simulink model "Backhoe_Arm_LS"  (R2013a)
settings: Solver=ode23t  StartTime=0.0  StopTime=30  MaxStep=0.01  RelTol=1e-3
PostLoadFcn:
  | warning off sm:compiler:state:UnsatisfiedDesiredTarget
  | warning off simscape:compiler:sli:init:SolverNotRecommended
  | warning off sm:sli:visualization:UnsupportedSimMode
  | warning off xPCTarget:sampleTime:sampleTimeInvariance
  | warning off sm:sli:setup:compile:LocalSolverNotSupported
model workspace (MAT data in the model file):
  cylinderGray = [0.6 0.6 0.6]
  darkOrange = [0.8 0.5 0]
  glassBlue = [0.2 0.2 1]
  gray = [0.3 0.3 0.3]
  orange = [0.8 0.65 0]
  pistonGray = [0.4 0.4 0.4]
  tireBlack = [0.1 0.1 0.1]
  wheelGray = [0.6 0.6 0.6]
  yellow = [0.8 0.8 0]
  rhoGlass = 2500
  rhoRubber = 1500
  rhoSteel = 7800
undefined symbols (not defined in the file or in its folder): BH_Param, sigbuilder_block, X, Y, Z
libraries: sm_lib x97, fl_lib x31, Backhoe_Lib x28, nesl_utility x21, sh_lib x9, xpclib x1
(part 1 of 4)
Description:
  | Copyright 2013 The MathWorks, Inc.
settings Model: ExtModeTrigDuration=3334  BufferReuse=off  Creator=smiller  LastModifiedBy=smiller
settings DataIOCC: LimitDataPoints=off
settings OptimizationCC: BlockReduction=off  OptimizeBlockIOStorage=off  BufferReuse=off  ExpressionFolding=off  ExpressionDepthLimit=2147483647  LocalBlockOutputs=off
settings DebuggingCC: SolverPrmCheckMsg=none
settings HardwareCC: ProdIntDivRoundTo=Zero  ProdEndianess=LittleEndian  ProdHWDeviceType=Generic->32-bit x86 compatible
settings RTWCC: SystemTargetFile=xpctarget.tlc  TemplateMakefile=xpc_default_tmf  Description=xPC Target  ProcessScript=xpctarget_make_rtw_hook  RTWCompilerOptimization=On
settings xpcTargetCC: TargetFcnLib=ansi_tfl_table_tmw.mat  CodeReplacementLibrary=XPC_BLAS  ParMdlRefBuildCompliant=on  ConcurrentExecutionCompliant=on  CombineSignalStateStructs=off  MATLABClassNameForMDSCustomization=xpcAperiodicCustomization  GRTInterface=on  GenerateAllocFcn=off  RL32LogBufSizeModifier=300000  xPCTaskExecutionProfile=off  xPCRL32EventNumber=5000  xPCLoadParamSetFile=off  xPCConcurrentTasks=off  xPCEnableSFAnimation=off
settings SimscapeCC: ExplicitSolverDiagnosticOptions=none
settings SimMechanicsCC: WarnOnRedundantConstraints=off
settings ExplorerConfigSet: InternalSimMechanicsExplorerSettings="<ExplorerConfiguration><canonicalview>default</canonicalview><TilePanel><TileInfo><Tiles Columns=\"1\" Count=\"1\" Rows=\"1\"><Column Left=\"2\" Weight=\"1\"/><Column Left=\"578\"/><Row Top=\"2\" Weight=\"1\"/><Row Top=\"405\"/><Tile Height=\"1\" Width=\"1\" X=\"0\" Y=\"0\"/></Tiles></TileInfo><SceneInfo><SceneViewer><BGColor><R>0.60000002384185791</R><G>0.60000002384185791</G><B>0.60000002384185791</B></BGColor><Camera><Position><X>19.674615884217218</X><Y>-11.790119899138375</Y><Z>8.3681328173355993</Z></Position><Center><X>1.1094029723013152</X><Y>-6.846774749183913</Y><Z>3.8240043455340573</Z></Center><Up><X>-0.20829119430312451</X><Y>0.11101192583651653</Y><Z>0.97174643333425503</Z></Up><Left>-4.3797052145004276</Left><Right>4.3797052145004276</Right><Bottom>-5.0912822484970093</Bottom><Top>5.0912822484970093</Top></Camera></SceneViewer></SceneInfo></TilePanel></ExplorerConfiguration>"

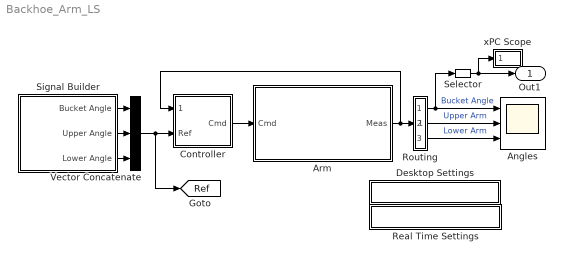
== system Backhoe_Arm_LS ==
  Angles : Scope  NumInputPorts=3
      settings: YMin=-120~-40~-70  YMax=20~60~-20
  Arm : Subsystem
      mask Display:
      | image(imread('Backhoe_Arm_IMAGE.JPG'));
      | port_label('input',1,'Cmd');
      | port_label('Output',1,'Meas');
  Controller : Subsystem
  Desktop Settings : Subsystem
      settings: OpenFcn=|
      | set_param(bdroot,'Solver','ODE23t','MaxStep','0.01','RelTol','1e-3','AbsTol','auto');
      | tvar_solverBlock = find_system(bdroot, 'SubClassName', 'solver');
      | 
      | for i=1:size(tvar_solverBlock,1)
      | 
      | set_param(char(tvar_solverBlock(i)), 'UseLocalSolver','off','DoFixedCost','off');
      | end
      | 
      | clear tvar_solverBlock
      mask Display: disp('Desktop Settings')
  Real Time Settings : Subsystem
      settings: OpenFcn=|
      | tvar_Nonlinear_Iterations = '2';
      | tvar_StepSize = '0.0004';                                                                                              %tvar_LocalSolver = 'NE_TRAPEZOIDAL_ADVANCER';
      | tvar_LocalSolver = 'NE_BACKWARD_EULER_ADVANCER';
      | set_param(bdroot,'Solver','ode1','FixedStep','auto');
      | tvar_solverBlock = find_system(bdroot, 'SubClassName', 'solver');
      | for i=1:size(tvar_solverBlock,1)
      | 
      | set_param(char(tvar_solverBlock(i)), 'UseLocalSolver','on','DoFixedCost','on','MaxNonlinIter',tvar_Nonlinear_Iterations,'LocalSolverChoice',tvar_LocalSolver,'LocalSolverSampleTime',tvar_StepSize);
      | end
      | clear tvar_Nonlinear_Iterations tvar_StepSize tvar_LocalSolver tvar_solverBlock
      mask Display: disp('Real Time Settings')
  Routing : Subsystem
  Selector : Selector  InputPortWidth=2  IndexOptions=Index vector (dialog)  Indices=[1]  OutputSizes=1
  Signal Builder : Subsystem  Tag=STV Subsys  LoadFcn=sigbuilder_block('load');  StartFcn=sigbuilder_block('start');  StopFcn=sigbuilder_block('stop');  ClipboardFcn=sigbuilder_block('clipboard');  mask(Sigbuilder block){}
      mask help: Simulink:masks:SigbuilderBlock_MD
      mask init:
      | if ~strcmp(get_param(bdroot(gcbh),'SimulationStatus'),'stopped') tuvar = sigbuilder_block('maskInit'); end
      settings: CopyFcn=sigbuilder_block('copy');  DeleteFcn=sigbuilder_block('delete');  ModelCloseFcn=sigbuilder_block('modelClose');  PreSaveFcn=sigbuilder_block('preSave');  PauseFcn=sigbuilder_block('pause');  ContinueFcn=sigbuilder_block('continue');  NameChangeFcn=sigbuilder_block('namechange');  OpenFcn=sigbuilder_block('open',[5.58621 7.44828 624.414 412.138 ]);  CloseFcn=sigbuilder_block('close');
      mask Display: plot(0, 0, 100, 100,[2, 2, 32, 32, 2], [68, 8, 8, 68, 68],[32, 2], [38, 38], [32, 19, 2],[53, 60, 44], [32, 17, 17, 2],[16, 16, 31, 31]);txt = getActiveGroup(gcbh);text(2, 100, txt,'verticalAlignment', 'top');
  Vector Concatenate : Concatenate  NumInputs=3
  xPC Scope : Subsystem
      mask Display: disp('xPC')
  Out1 : Outport
  tag scope: Ref=global
  wires:
  Signal Builder/2(Upper Angle) -> Vector Concatenate/2
  Signal Builder/1(Bucket Angle) -> Vector Concatenate/1
  Signal Builder/3(Lower Angle) -> Vector Concatenate/3
  Vector Concatenate/1 -> [Ref], Controller/2(Ref)
  Arm/1(Meas) -> Controller/1(Meas), Routing/1(Meas)
  Controller/1(Cmd) -> Arm/1(Cmd)
  Routing/2(UArm) -> Angles/2  "Upper Arm"
  Routing/3(LArm) -> Angles/3  "Lower Arm"
  Routing/1(Bucket) -> Angles/1, Selector/1  "Bucket Angle"
  Selector/1 -> xPC Scope/1(In1), Out1/1

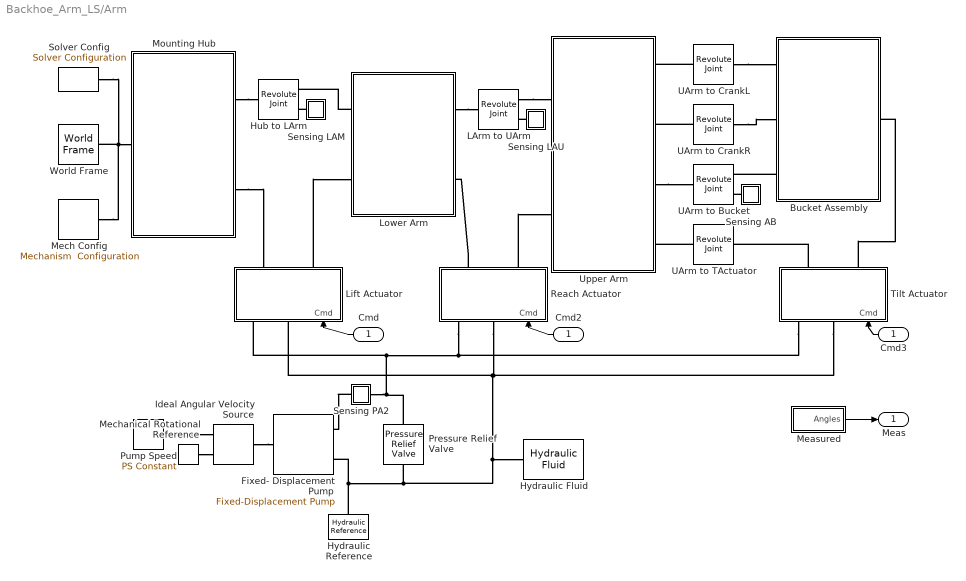
== system Backhoe_Arm_LS/Arm ==
  Cmd : Inport
  Bucket Assembly : Subsystem
      mask Display:
      | image(imread('Backhoe_Arm_Bucket_Asy_IMAGE.JPG'));
      | port_label('lconn',1,'UAL');
      | port_label('lconn',2,'UAR');
      | port_label('lconn',3,'UA');
      | port_label('rconn',1,'TAct');
  Cmd2 : InportShadow
  Cmd3 : InportShadow
  Fixed- Displacement Pump : sh_lib/Pumps and Motors/Fixed-Displacement Pump  D=BH_Param.Hydraulic.Pump.Displacement m^3/rad  efficiency_vol=BH_Param.Hydraulic.Pump.Vol_Eff  efficiency_tot=BH_Param.Hydraulic.Pump.Total_Eff  pr_nominal=BH_Param.Hydraulic.Pump.Nominal_Pressure Pa  w_nominal=BH_Param.Hydraulic.Pump.Nominal_Ang_Vel rad/s  visc_nominal=BH_Param.Hydraulic.Pump.Nominal_Kin_Visc cSt  pump_delivery_Log=off  leakage_flow_Log=off  torque_Log=off  power_hyd_Log=off  pressure_diff_Log=off  shaft_ang_vel_Log=off  LocalVarNames=|pump_delivery|leakage_flow|torque|power_hyd|pressure_diff|shaft_ang_vel  LocalVarDescs=|Pump delivery (m^3/s)|Leakage flow rate (m^3/s)|Driving shaft torque (N*m)|Output flow power (W)|Pressure differential (Pa)|Driving shaft angular velocity (rad/s)  LocalVarLogging=[0 0 0 0 0 0]
  Hub to LArm : sm_lib/Joints/Revolute Joint  SenseConstraintForceX=off  SenseConstraintForceY=off  SenseConstraintForceZ=off  SenseConstraintTorqueX=off  SenseConstraintTorqueY=off  SenseConstraintTorqueZ=off  ConstraintWrenchDir=FollowerOnBase  ConstraintWrenchFrame=BaseFrame  EquilibriumPosition=0  EquilibriumPositionUnits=deg  SpringStiffness=0  SpringStiffnessUnits=N*m/deg  DampingCoefficient=0  DampingCoefficientUnits=N*m/(deg/s)  ActuationMode=NoActuation  SensePosition=on  SenseVelocity=off  SenseAcceleration=off  SenseTorqueForce=off  PositionTargetValue=-60  PositionTargetValueUnits=deg  PositionTargetSpecify=on  PositionTargetPriority=High  VelocityTargetValue=0  VelocityTargetValueUnits=deg/s  VelocityTargetSpecify=off  VelocityTargetPriority=High  BlockFunction=simmechanics.library.joints.revolute_joint
  Hydraulic Reference : fl_lib/Hydraulic/Hydraulic Elements/Hydraulic Reference  q_Log=off  LocalVarNames=|q  LocalVarDescs=|q  LocalVarLogging=[]
  Hydraulic Fluid : sh_lib/Hydraulic Utilities/Hydraulic Fluid  Tag=Factory Generic  DataSource=1  SelFluid=9  SysTemp=50 c  TrapAir=0.004  ViscDerFactor=1  LocalVarLogging=[]
  Ideal Angular Velocity Source : fl_lib/Mechanical/Mechanical Sources/Ideal Angular Velocity Source  w_Log=off  t_Log=off  LocalVarNames=|torque|rel_velocity|power  LocalVarDescs=|Torque (N*m)|Relative velocity (rad/s)|Power generated by the sourcec(W)  LocalVarLogging=[0 0 0]
  LArm to UArm : sm_lib/Joints/Revolute Joint  SenseConstraintForceX=off  SenseConstraintForceY=off  SenseConstraintForceZ=off  SenseConstraintTorqueX=off  SenseConstraintTorqueY=off  SenseConstraintTorqueZ=off  ConstraintWrenchDir=FollowerOnBase  ConstraintWrenchFrame=BaseFrame  EquilibriumPosition=0  EquilibriumPositionUnits=deg  SpringStiffness=0  SpringStiffnessUnits=N*m/deg  DampingCoefficient=0  DampingCoefficientUnits=N*m/(deg/s)  ActuationMode=NoActuation  SensePosition=on  SenseVelocity=off  SenseAcceleration=off  SenseTorqueForce=off  PositionTargetValue=50  PositionTargetValueUnits=deg  PositionTargetSpecify=on  PositionTargetPriority=High  VelocityTargetValue=0  VelocityTargetValueUnits=deg/s  VelocityTargetSpecify=off  VelocityTargetPriority=High  BlockFunction=simmechanics.library.joints.revolute_joint
  Lift Actuator : Subsystem  mask(Hydraulic Actuator){Lcyl=BH_Param.Lift_Actuator.Cyl_Dims.Lcyl, Rcyl=BH_Param.Lift_Actuator.Cyl_Dims.Rcyl, Lbase=BH_Param.Lift_Actuator.Cyl_Dims.Lbase, Wbase=BH_Param.Lift_Actuator.Cyl_Dims.Wbase, Rbp=BH_Param.Lift_Actuator.Cyl_Dims.Rbp, Lbp=BH_Param.Lift_Actuator.Cyl_Dims.Lbp, Lpist=BH_Param.Lift_Actuator.Piston_Dims.Lpist, Rpist=BH_Param.Lift_Actuator.Piston_Dims.Rpist, Whead=BH_Param.Lift_Actuator.Piston_Dims.Whead, Lhead=BH_Param.Lift_Actuator.Piston_Dims.Lhead, Rhp=BH_Param.Lift_Actuator.Piston_Dims.Rhp, Lhp=BH_Param.Lift_Actuator.Piston_Dims.Lhp, hydr_area=BH_Param.Lift_Actuator.Cylinder.Area_A, hydr_stroke=BH_Param.Lift_Actuator.Cylinder.Stroke, hydr_deadvol=BH_Param.Lift_Actuator.Cylinder.DeadVol_A, hydr_x0=BH_Param.Lift_Actuator.Cylinder.x0, hydr_PA0=BH_Param.Lift_Actuator.Cylinder.PA0, hydr_PB0=BH_Param.Lift_Actuator.Cylinder.PB0, hydr_valve_max_area=BH_Param.Lift_Actuator.Valve.Max_Area, hydr_valve_max_opening=BH_Param.Lift_Actuator.Valve.Max_Opening, friction_breakaway=BH_Param.Lift_Actuator.Friction.Breakaway, friction_coulomb=BH_Param.Lift_Actuator.Friction.Coulomb, friction_viscous=BH_Param.Lift_Actuator.Friction.Viscous, circlePoints=25, cylColor=BH_Param.Colors.cylinderGray, rhoCyl=BH_Param.Densities.rhoSteel, pistColor=BH_Param.Colors.pistonGray, rhoPist=BH_Param.Densities.rhoSteel, connColor=BH_Param.Colors.gray, rhoConn=BH_Param.Densities.rhoSteel}
      mask prompts: Lcyl "Lcyl [m]"; Rcyl "Rcyl [m]"; Lbase "Lbase [m]"; Wbase "Wbase [m]"; Rbp "Rbp [m]"; Lbp "Lbp [m]"; Lpist "Lpist [m]"; Rpist "Rpist [m]"; Whead "Whead [m]"; Lhead "Lhead [m]"; Rhp "Rhp [m]"; Lhp "Lhp [m]"; hydr_area "Piston Area [m^3]"; hydr_stroke "Piston Stroke [m]"; hydr_deadvol "Dead Volume [m^3]"; hydr_x0 "Initial Position [m]"; hydr_PA0 "Initial Pressure, Chamber A [Pa]"; hydr_PB0 "Initial Pressure, Chamber B [Pa]"; hydr_valve_max_area "Valve Max Area [mm^2]"; hydr_valve_max_opening "Valve Max Opening [m]"; friction_breakaway "Breakaway Friction Force [N]"; friction_coulomb "Coulomb Friction Force [N]"; friction_viscous "Viscous Friction Coefficient [N/(m/2)]"; circlePoints "Circle Mesh Resolution"; cylColor "Cylinder Color"; rhoCyl "Cylinder Density [kg/m^3]"; pistColor "Piston Color"; rhoPist "Piston Density [kg/m^3]"; connColor "Connector Color"; rhoConn "Connector Density [kg/m^3]"
      mask help:
      | Consists of the backhoe hydraulic actuator assembly.
      |
      | Zero piston displacement corresponds to the piston and cylinder centers of mass in the same position. Positive piston displacement is outward motion, and negative piston displacement is inward motion.
      |
      | Attachment points are:
      | C: Center of the Cylinder base bracket hole.
      | H: Center of the Piston Head bracket hole.
      | Both attachment points are configured for Revolute joints.
      |
      | The Simulink Signal input port supplies a Pressure value P (in Pa) to a Simscape hydraulic network.
      |
      | Click on Help to view a schematic of the hydraulic actuator, its configurable dimension parameters and attachment points (in red).
      mask init:
      | % Hollow Cylinder cross-section
      | cylSection = [];
      | 
      | for i = 0:2*circlePoints
      |     angle = (i/circlePoints)*pi;
      |     cylSection = [cylSection; Rcyl*cos(angle) Rcyl*sin(angle)];
      | end
      | 
      | for i = 0:2*circlePoints
      |     angle = -(i/circlePoints)*pi;
      |     cylSection = [cylSection; Rpist*cos(angle) Rpist*sin(angle)];
      | end
      mask Help: web('Backhoe_Actuator.html');
      mask Display:
      | image(imread('Backhoe_Arm_Actuator_IMAGE.jpg'));
      | port_label('lconn',1,'T');
      | port_label('lconn',2,'P');
      | port_label('rconn',1,'LA');
      | port_label('rconn',2,'H');
      | port_label('input',1,'Cmd');
  "Lower Arm " : Subsystem
      mask Display:
      | image(imread('Backhoe_Arm_Lower_IMAGE.JPG'));
      | port_label('lconn',1,'H');
      | port_label('lconn',2,'LAct');
      | port_label('rconn',1,'UA');
      | port_label('rconn',2,'RAct');
  Measured : Subsystem
  Mech Config : sm_lib/Utilities/Mechanism  Configuration  GravityVector=[0 0 -9.81]  GravityUnits=m/s^2  AllowGravitySignal=off  LinearizationDelta=0.001  BlockFunction=simmechanics.library.utilities.mechanism_configuration
  Mechanical Rotational Reference : fl_lib/Mechanical/Rotational Elements/Mechanical Rotational Reference  t_Log=off  LocalVarNames=|t  LocalVarDescs=|t  LocalVarLogging=[]
  Mounting Hub : Subsystem  mask(Mounting Hub){Hleft=1, Hright=2, Ltop=0.75, Lbottom=1.5, Tplate=0.3, Dplates=1.2, plateFillet=0.25, numPoints=15, L1=0.75, H1=0.25, RH1=0.075, L2=0.75, H2=1.75, RH2=0.075, L3=0.5, H3=0.5, Larm=0.8, Warm=0.5, Tarm=0.5, Tab=0.1, RH3=0.075, Dbracket=1.1, Lbracket=1.2, Wbracket=1.2, Tbracket=2, Hbracket=1, Rhole=0.1, Hhole=0.5, hubColor=orange, rho=rhoSteel}
      mask prompts: Hleft "Hleft [m]"; Hright "Hright [m]"; Ltop "Ltop [m]"; Lbottom "Lbottom [m]"; Tplate "Tplate [m]"; Dplates "Dplates [m]"; plateFillet "Plate Fillet Radius [m]"; numPoints "Fillet Point Resolution"; L1 "L1 [m]"; H1 "H1 [m]"; RH1 "RH1 [m]"; L2 "L2 [m]"; H2 "H2 [m]"; RH2 "RH2 [m]"; L3 "L3 [m]"; H3 "H3 [m]"; Larm "Larm [m]"; Warm "Warm [m]"; Tarm "Tarm [m]"; Tab "Tab [m]"; RH3 "RH3 [m]"; Dbracket "Dbracket [m]"; Lbracket "Lbracket [m]"; Wbracket "Wbracket [m]"; Tbracket "Tbracket [m]"; Hbracket "Hbracket [m]"; Rhole "Rhole [m]"; Hhole "Hhole [m]"; hubColor "Hub Color"; rho "Density [kg/m^3]"
      mask help:
      | Consists of the backhoe mounting hub assembly.
      |
      | This assembly connects to the Backhoe Arm assembly on the front end, and to the Mounting Base assembly on the rear and side.
      |
      | Attachment points are:
      | LH: Left base hydraulic actuator (piston Head).
      | RH: Right base hydraulic actuator (piston Head).
      | LC: Lower arm hydraulic actuator (Cylinder base).
      | LA: Lower Arm joint.
      | MB: Mounting Base joint.
      | All attachments are configured for Revolute Joints.
      |
      | Click on Help to view a schematic of the bracket, its configurable dimension parameters and attachment points (in red).
      mask init:
      | plateSection = [0              0     ; ...
      |                 Lbottom        0     ; ...
      |                 Lbottom        Hright; ...
      |                 (Lbottom-Ltop) Hright; ...
      |                 0              Hleft];
      | plateSection = Extr_Data_Round_Corners(plateSection,1:5,0.1,15);
      mask Help: web('Backhoe_Mountinghub.html');
      mask Display:
      | image(imread('Backhoe_Arm_Base_IMAGE.JPG'));
      | port_label('lconn',1,'B');
      | port_label('rconn',1,'LArm');
      | port_label('rconn',2,'LAct');
  Pressure Relief Valve : sh_lib/Valves/Pressure Control Valves/Pressure Relief Valve  area_max=BH_Param.Hydraulic.PRV.Max_Area m^2  pres_set=BH_Param.Hydraulic.PRV.Pressure_Set Pa  reg_range=BH_Param.Hydraulic.PRV.Pressure_Rng Pa  C_d=BH_Param.Hydraulic.PRV.Flow_Disch_Coeff  Re_cr=BH_Param.Hydraulic.PRV.Re_Critical  A_leak=BH_Param.Hydraulic.PRV.Leakage_Area m^2  flow_rate_Log=off  pr_drop_Log=off  power_Log=off  area_Log=off  Re_Log=off  LocalVarNames=|flow_rate|pr_drop|power|area|Re  LocalVarDescs=|Flow rate through the valve (m^3/s)|Pressure differential across the valve (Pa)|Hydraulic loss power (W)|Instantaneous passage area (m^2)|Reynolds number  LocalVarLogging=[0 0 0 0 0]
  Pump Speed : fl_lib/Physical Signals/Sources/PS Constant  constant=BH_Param.Hydraulic.Pump.Speed  LocalVarLogging=[]
  Reach Actuator : Subsystem  mask(Hydraulic Actuator){Lcyl=BH_Param.Reach_Actuator.Cyl_Dims.Lcyl, Rcyl=BH_Param.Reach_Actuator.Cyl_Dims.Rcyl, Lbase=BH_Param.Reach_Actuator.Cyl_Dims.Lbase, Wbase=BH_Param.Reach_Actuator.Cyl_Dims.Wbase, Rbp=BH_Param.Reach_Actuator.Cyl_Dims.Rbp, Lbp=BH_Param.Reach_Actuator.Cyl_Dims.Lbp, Lpist=BH_Param.Reach_Actuator.Piston_Dims.Lpist, Rpist=BH_Param.Reach_Actuator.Piston_Dims.Rpist, Whead=BH_Param.Reach_Actuator.Piston_Dims.Whead, Lhead=BH_Param.Reach_Actuator.Piston_Dims.Lhead, Rhp=BH_Param.Reach_Actuator.Piston_Dims.Rhp, Lhp=BH_Param.Reach_Actuator.Piston_Dims.Lhp, hydr_area=BH_Param.Reach_Actuator.Cylinder.Area_A, hydr_stroke=BH_Param.Reach_Actuator.Cylinder.Stroke, hydr_deadvol=BH_Param.Reach_Actuator.Cylinder.DeadVol_A, hydr_x0=BH_Param.Reach_Actuator.Cylinder.x0, hydr_PA0=BH_Param.Reach_Actuator.Cylinder.PA0, hydr_PB0=BH_Param.Reach_Actuator.Cylinder.PB0, hydr_valve_max_area=BH_Param.Reach_Actuator.Valve.Max_Area, hydr_valve_max_opening=BH_Param.Reach_Actuator.Valve.Max_Opening, friction_breakaway=BH_Param.Reach_Actuator.Friction.Breakaway, friction_coulomb=BH_Param.Reach_Actuator.Friction.Coulomb, friction_viscous=BH_Param.Reach_Actuator.Friction.Viscous, circlePoints=25, cylColor=BH_Param.Colors.cylinderGray, rhoCyl=BH_Param.Densities.rhoSteel, pistColor=BH_Param.Colors.pistonGray, rhoPist=BH_Param.Densities.rhoSteel, connColor=BH_Param.Colors.gray, rhoConn=BH_Param.Densities.rhoSteel}
      mask prompts: Lcyl "Lcyl [m]"; Rcyl "Rcyl [m]"; Lbase "Lbase [m]"; Wbase "Wbase [m]"; Rbp "Rbp [m]"; Lbp "Lbp [m]"; Lpist "Lpist [m]"; Rpist "Rpist [m]"; Whead "Whead [m]"; Lhead "Lhead [m]"; Rhp "Rhp [m]"; Lhp "Lhp [m]"; hydr_area "Piston Area [m^3]"; hydr_stroke "Piston Stroke [m]"; hydr_deadvol "Dead Volume [m^3]"; hydr_x0 "Initial Position [m]"; hydr_PA0 "Initial Pressure, Chamber A [Pa]"; hydr_PB0 "Initial Pressure, Chamber B [Pa]"; hydr_valve_max_area "Valve Max Area [mm^2]"; hydr_valve_max_opening "Valve Max Opening [m]"; friction_breakaway "Breakaway Friction Force [N]"; friction_coulomb "Coulomb Friction Force [N]"; friction_viscous "Viscous Friction Coefficient [N/(m/2)]"; circlePoints "Circle Mesh Resolution"; cylColor "Cylinder Color"; rhoCyl "Cylinder Density [kg/m^3]"; pistColor "Piston Color"; rhoPist "Piston Density [kg/m^3]"; connColor "Connector Color"; rhoConn "Connector Density [kg/m^3]"
      mask help:
      | Consists of the backhoe hydraulic actuator assembly.
      |
      | Zero piston displacement corresponds to the piston and cylinder centers of mass in the same position. Positive piston displacement is outward motion, and negative piston displacement is inward motion.
      |
      | Attachment points are:
      | C: Center of the Cylinder base bracket hole.
      | H: Center of the Piston Head bracket hole.
      | Both attachment points are configured for Revolute joints.
      |
      | The Simulink Signal input port supplies a Pressure value P (in Pa) to a Simscape hydraulic network.
      |
      | Click on Help to view a schematic of the hydraulic actuator, its configurable dimension parameters and attachment points (in red).
      mask init: same as Backhoe_Arm_LS/Arm/Lift Actuator
      mask Help: web('Backhoe_Actuator.html');
      mask Display:
      | image(imread('Backhoe_Arm_Actuator_IMAGE.jpg'));
      | port_label('lconn',1,'T');
      | port_label('lconn',2,'P');
      | port_label('rconn',1,'UA');
      | port_label('rconn',2,'LA');
      | port_label('input',1,'Cmd');
  Sensing AB : Subsystem
      mask Display: disp('S')
  Sensing LAM : Subsystem
      mask Display: disp('S')
  Sensing LAU : Subsystem
      mask Display: disp('S')
  Sensing PA2 : Subsystem
      mask Display: disp('S')
  Solver Config : nesl_utility/Solver Configuration  PhysicalDomain=network_engine_domain  SubClassName=solver  LeftPortType=input  RightPortType=generic  Accelerate=off  Tones=[]  Harmonics=[]  SimulateNoise=off  Profile=off  UseLocalSampling=off  EnableSwitchedLinearOptims=on  FrequencyDomain=off  UseCCode=off  UseNewInitialization=off  DoDC=off  ResidualTolerance=1e-9  UseLocalSolver=off  LocalSolverChoice=NE_BACKWARD_EULER_ADVANCER  LocalSolverSampleTime=0.0004  DoFixedCost=off  MaxNonlinIter=2  MaxModeIter=2  LinearAlgebra=Sparse  DelaysMemoryBudget=1024
  Tilt Actuator : Subsystem  mask(Hydraulic Actuator){Lcyl=BH_Param.Tilt_Actuator.Cyl_Dims.Lcyl, Rcyl=BH_Param.Tilt_Actuator.Cyl_Dims.Rcyl, Lbase=BH_Param.Tilt_Actuator.Cyl_Dims.Lbase, Wbase=BH_Param.Tilt_Actuator.Cyl_Dims.Wbase, Rbp=BH_Param.Tilt_Actuator.Cyl_Dims.Rbp, Lbp=BH_Param.Tilt_Actuator.Cyl_Dims.Lbp, Lpist=BH_Param.Tilt_Actuator.Piston_Dims.Lpist, Rpist=BH_Param.Tilt_Actuator.Piston_Dims.Rpist, Whead=BH_Param.Tilt_Actuator.Piston_Dims.Whead, Lhead=BH_Param.Tilt_Actuator.Piston_Dims.Lhead, Rhp=BH_Param.Tilt_Actuator.Piston_Dims.Rhp, Lhp=BH_Param.Tilt_Actuator.Piston_Dims.Lhp, hydr_area=BH_Param.Tilt_Actuator.Cylinder.Area_A, hydr_stroke=BH_Param.Tilt_Actuator.Cylinder.Stroke, hydr_deadvol=BH_Param.Tilt_Actuator.Cylinder.DeadVol_A, hydr_x0=BH_Param.Tilt_Actuator.Cylinder.x0, hydr_PA0=BH_Param.Tilt_Actuator.Cylinder.PA0, hydr_PB0=BH_Param.Tilt_Actuator.Cylinder.PB0, hydr_valve_max_area=BH_Param.Tilt_Actuator.Valve.Max_Area, hydr_valve_max_opening=BH_Param.Tilt_Actuator.Valve.Max_Opening, friction_breakaway=BH_Param.Tilt_Actuator.Friction.Breakaway, friction_coulomb=BH_Param.Tilt_Actuator.Friction.Coulomb, friction_viscous=BH_Param.Tilt_Actuator.Friction.Viscous, circlePoints=25, cylColor=BH_Param.Colors.cylinderGray, rhoCyl=BH_Param.Densities.rhoSteel, pistColor=BH_Param.Colors.pistonGray, rhoPist=BH_Param.Densities.rhoSteel, connColor=BH_Param.Colors.gray, rhoConn=BH_Param.Densities.rhoSteel}
      mask prompts: Lcyl "Lcyl [m]"; Rcyl "Rcyl [m]"; Lbase "Lbase [m]"; Wbase "Wbase [m]"; Rbp "Rbp [m]"; Lbp "Lbp [m]"; Lpist "Lpist [m]"; Rpist "Rpist [m]"; Whead "Whead [m]"; Lhead "Lhead [m]"; Rhp "Rhp [m]"; Lhp "Lhp [m]"; hydr_area "Piston Area [m^3]"; hydr_stroke "Piston Stroke [m]"; hydr_deadvol "Dead Volume [m^3]"; hydr_x0 "Initial Position [m]"; hydr_PA0 "Initial Pressure, Chamber A [Pa]"; hydr_PB0 "Initial Pressure, Chamber B [Pa]"; hydr_valve_max_area "Valve Max Area [mm^2]"; hydr_valve_max_opening "Valve Max Opening [m]"; friction_breakaway "Breakaway Friction Force [N]"; friction_coulomb "Coulomb Friction Force [N]"; friction_viscous "Viscous Friction Coefficient [N/(m/2)]"; circlePoints "Circle Mesh Resolution"; cylColor "Cylinder Color"; rhoCyl "Cylinder Density [kg/m^3]"; pistColor "Piston Color"; rhoPist "Piston Density [kg/m^3]"; connColor "Connector Color"; rhoConn "Connector Density [kg/m^3]"
      mask help:
      | Consists of the backhoe hydraulic actuator assembly.
      |
      | Zero piston displacement corresponds to the piston and cylinder centers of mass in the same position. Positive piston displacement is outward motion, and negative piston displacement is inward motion.
      |
      | Attachment points are:
      | C: Center of the Cylinder base bracket hole.
      | H: Center of the Piston Head bracket hole.
      | Both attachment points are configured for Revolute joints.
      |
      | The Simulink Signal input port supplies a Pressure value P (in Pa) to a Simscape hydraulic network.
      |
      | Click on Help to view a schematic of the hydraulic actuator, its configurable dimension parameters and attachment points (in red).
      mask init: same as Backhoe_Arm_LS/Arm/Lift Actuator
      mask Help: web('Backhoe_Actuator.html');
      mask Display:
      | image(imread('Backhoe_Arm_Actuator_IMAGE.jpg'));
      | port_label('lconn',1,'T');
      | port_label('lconn',2,'P');
      | port_label('rconn',1,'UA');
      | port_label('rconn',2,'LA');
      | port_label('input',1,'Cmd');
  UArm to Bucket : sm_lib/Joints/Revolute Joint  SenseConstraintForceX=off  SenseConstraintForceY=off  SenseConstraintForceZ=off  SenseConstraintTorqueX=off  SenseConstraintTorqueY=off  SenseConstraintTorqueZ=off  ConstraintWrenchDir=FollowerOnBase  ConstraintWrenchFrame=BaseFrame  EquilibriumPosition=0  EquilibriumPositionUnits=deg  SpringStiffness=0  SpringStiffnessUnits=N*m/deg  DampingCoefficient=0  DampingCoefficientUnits=N*m/(deg/s)  ActuationMode=NoActuation  SensePosition=on  SenseVelocity=off  SenseAcceleration=off  SenseTorqueForce=off  PositionTargetValue=0  PositionTargetValueUnits=deg  PositionTargetSpecify=on  PositionTargetPriority=High  VelocityTargetValue=0  VelocityTargetValueUnits=deg/s  VelocityTargetSpecify=off  VelocityTargetPriority=High  BlockFunction=simmechanics.library.joints.revolute_joint
  UArm to CrankL : sm_lib/Joints/Revolute Joint  SenseConstraintForceX=off  SenseConstraintForceY=off  SenseConstraintForceZ=off  SenseConstraintTorqueX=off  SenseConstraintTorqueY=off  SenseConstraintTorqueZ=off  ConstraintWrenchDir=FollowerOnBase  ConstraintWrenchFrame=BaseFrame  EquilibriumPosition=0  EquilibriumPositionUnits=deg  SpringStiffness=0  SpringStiffnessUnits=N*m/deg  DampingCoefficient=0  DampingCoefficientUnits=N*m/(deg/s)  ActuationMode=NoActuation  SensePosition=off  SenseVelocity=off  SenseAcceleration=off  SenseTorqueForce=off  PositionTargetValue=-150  PositionTargetValueUnits=deg  PositionTargetSpecify=off  PositionTargetPriority=Low  VelocityTargetValue=0  VelocityTargetValueUnits=deg/s  VelocityTargetSpecify=off  VelocityTargetPriority=High  BlockFunction=simmechanics.library.joints.revolute_joint
  UArm to CrankR : sm_lib/Joints/Revolute Joint  SenseConstraintForceX=off  SenseConstraintForceY=off  SenseConstraintForceZ=off  SenseConstraintTorqueX=off  SenseConstraintTorqueY=off  SenseConstraintTorqueZ=off  ConstraintWrenchDir=FollowerOnBase  ConstraintWrenchFrame=BaseFrame  EquilibriumPosition=0  EquilibriumPositionUnits=deg  SpringStiffness=0  SpringStiffnessUnits=N*m/deg  DampingCoefficient=0  DampingCoefficientUnits=N*m/(deg/s)  ActuationMode=NoActuation  SensePosition=off  SenseVelocity=off  SenseAcceleration=off  SenseTorqueForce=off  PositionTargetValue=0  PositionTargetValueUnits=deg  PositionTargetSpecify=off  PositionTargetPriority=High  VelocityTargetValue=0  VelocityTargetValueUnits=deg/s  VelocityTargetSpecify=off  VelocityTargetPriority=High  BlockFunction=simmechanics.library.joints.revolute_joint
  UArm to TActuator : sm_lib/Joints/Revolute Joint  SenseConstraintForceX=off  SenseConstraintForceY=off  SenseConstraintForceZ=off  SenseConstraintTorqueX=off  SenseConstraintTorqueY=off  SenseConstraintTorqueZ=off  ConstraintWrenchDir=FollowerOnBase  ConstraintWrenchFrame=BaseFrame  EquilibriumPosition=0  EquilibriumPositionUnits=deg  SpringStiffness=0  SpringStiffnessUnits=N*m/deg  DampingCoefficient=0  DampingCoefficientUnits=N*m/(deg/s)  ActuationMode=NoActuation  SensePosition=off  SenseVelocity=off  SenseAcceleration=off  SenseTorqueForce=off  PositionTargetValue=-90  PositionTargetValueUnits=deg  PositionTargetSpecify=on  PositionTargetPriority=Low  VelocityTargetValue=0  VelocityTargetValueUnits=deg/s  VelocityTargetSpecify=off  VelocityTargetPriority=High  BlockFunction=simmechanics.library.joints.revolute_joint
  Upper Arm : Subsystem
      mask Display:
      | image(imread('Backhoe_Arm_Upper_IMAGE.JPG'));
      | port_label('lconn',1,'LA');
      | port_label('lconn',2,'RAct');
      | port_label('rconn',1,'CrL');
      | port_label('rconn',2,'CrR');
      | port_label('rconn',3,'B');
      | port_label('rconn',4,'TAct');
  World Frame : sm_lib/Frames and  Transforms/World Frame  BlockFunction=simmechanics.library.frames_transforms.world_frame
  Meas : Outport
  wires:
  Cmd3/1 -> Tilt Actuator/1(Cmd)
  Cmd2/1 -> Reach Actuator/1(Cmd)
  Measured/1(Angles) -> Meas/1
  Cmd/1 -> Lift Actuator/1(Cmd)
  connections:
  Reach Actuator/RConn2 -- "Lower Arm "/RConn2
  Upper Arm/RConn3 -- UArm to Bucket/LConn1
  "Lower Arm "/RConn1 -- LArm to UArm/LConn1
  Mech Config/RConn1 -- Mounting Hub/LConn1 -- Solver Config/RConn1 -- World Frame/RConn1
  "Lower Arm "/LConn1 -- Hub to LArm/RConn1
  Lift Actuator/RConn1 -- "Lower Arm "/LConn2
  Mounting Hub/RConn1 -- Hub to LArm/LConn1
  LArm to UArm/RConn1 -- Upper Arm/LConn1
  Reach Actuator/RConn1 -- Upper Arm/LConn2
  UArm to CrankR/LConn1 -- Upper Arm/RConn2
  UArm to CrankL/LConn1 -- Upper Arm/RConn1
  Sensing LAM/LConn1 -- Hub to LArm/RConn2
  Sensing LAU/LConn1 -- LArm to UArm/RConn2
  Sensing AB/LConn1 -- UArm to Bucket/RConn2
  Tilt Actuator/RConn1 -- Bucket Assembly/RConn1
  UArm to CrankL/RConn1 -- Bucket Assembly/LConn1
  UArm to CrankR/RConn1 -- Bucket Assembly/LConn2
  Bucket Assembly/LConn3 -- UArm to Bucket/RConn1
  Mounting Hub/RConn2 -- Lift Actuator/RConn2
  UArm to TActuator/LConn1 -- Upper Arm/RConn4
  Tilt Actuator/RConn2 -- UArm to TActuator/RConn1
  Pressure Relief Valve/LConn1 -- Tilt Actuator/LConn2 -- Reach Actuator/LConn2 -- Lift Actuator/LConn2 -- Sensing PA2/RConn1
  Pressure Relief Valve/RConn1 -- Hydraulic Fluid/RConn1 -- Lift Actuator/LConn1 -- Tilt Actuator/LConn1 -- Reach Actuator/LConn1 -- Hydraulic Reference/LConn1 -- Fixed- Displacement Pump/RConn2
  Pump Speed/RConn1 -- Ideal Angular Velocity Source/RConn1
  Ideal Angular Velocity Source/LConn1 -- Fixed- Displacement Pump/LConn1
  Mechanical Rotational Reference/LConn1 -- Ideal Angular Velocity Source/RConn2
  Sensing PA2/LConn1 -- Fixed- Displacement Pump/RConn1

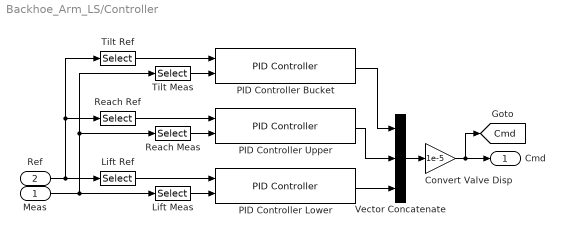
== system Backhoe_Arm_LS/Controller ==
  Meas : Inport
  Ref : Inport  Port=2
  Convert Valve Disp : Gain  Gain=1e-5
  Lift Meas : Selector  InputPortWidth=3  IndexOptions=Index vector (dialog)  Indices=3  OutputSizes=1
  Lift Ref : Selector  InputPortWidth=3  IndexOptions=Index vector (dialog)  Indices=3  OutputSizes=1
  PID Controller Bucket : Backhoe_Lib/PID Controller  upperLim=10  lowerLim=-120  Kp=10  Ki=0.01  Kd=0.01  N=100
  PID Controller Lower : Backhoe_Lib/PID Controller  upperLim=40  lowerLim=-70  Kp=30  Ki=0.002  Kd=0.002  N=100
  PID Controller Upper : Backhoe_Lib/PID Controller  upperLim=60  lowerLim=-20  Kp=24  Ki=0  Kd=0  N=100
  Reach Meas : Selector  InputPortWidth=3  IndexOptions=Index vector (dialog)  Indices=2  OutputSizes=1
  Reach Ref : Selector  InputPortWidth=3  IndexOptions=Index vector (dialog)  Indices=2  OutputSizes=1
  "Tilt Meas " : Selector  InputPortWidth=3  IndexOptions=Index vector (dialog)  Indices=1  OutputSizes=1
  Tilt Ref : Selector  InputPortWidth=3  IndexOptions=Index vector (dialog)  Indices=1  OutputSizes=1
  Vector Concatenate : Concatenate  NumInputs=3
  Cmd : Outport
  tag scope: Cmd=global
  wires:
  "Tilt Meas "/1 -> PID Controller Bucket/2
  Tilt Ref/1 -> PID Controller Bucket/1
  Reach Meas/1 -> PID Controller Upper/2
  Reach Ref/1 -> PID Controller Upper/1
  Lift Ref/1 -> PID Controller Lower/1
  Lift Meas/1 -> PID Controller Lower/2
  Meas/1 -> "Tilt Meas "/1, Reach Meas/1, Lift Meas/1
  Ref/1 -> Lift Ref/1, Tilt Ref/1, Reach Ref/1
  Vector Concatenate/1 -> Convert Valve Disp/1
  Convert Valve Disp/1 -> Cmd/1, [Cmd]
  PID Controller Upper/1 -> Vector Concatenate/2
  PID Controller Lower/1 -> Vector Concatenate/3
  PID Controller Bucket/1 -> Vector Concatenate/1

== system Backhoe_Arm_LS/Desktop Settings ==

== system Backhoe_Arm_LS/Real Time Settings ==

== system Backhoe_Arm_LS/Routing ==
  Meas : Inport
  Demux : Demux  Outputs=3
  Demux1 : Demux  Outputs=3
  Mux : Mux  Inputs=2
  Mux1 : Mux  Inputs=2
  Mux2 : Mux  Inputs=2
  Bucket : Outport
  UArm : Outport  Port=2
  LArm : Outport  Port=3
  wires:
  Demux/3 -> Mux/1
  Demux/2 -> Mux1/1
  Demux1/1 -> Mux2/2
  Mux/1 -> LArm/1  "Lower Arm"
  Mux1/1 -> UArm/1  "Upper Arm"
  Demux/1 -> Mux2/1
  Demux1/3 -> Mux/2
  Demux1/2 -> Mux1/2
  Mux2/1 -> Bucket/1  "Bucket"
  [Ref] -> Demux1/1
  Meas/1 -> Demux/1

== system Backhoe_Arm_LS/Signal Builder ==
  Demux : Demux  Tag=STV Demux  Outputs=3
  FromWs : FromWorkspace  Tag=STV FromWs  VariableName=tuvar  SampleTime=0  OutputAfterFinalValue=Holding final value
      SigBuilderData=|
      | common.afterFinalStr = 'Hold final value'
      | common.sampleTime = '0'
      | dataSet.timeRange = [0 60]
      | dataSet.name = 'Ref'
      | sbobj.Groups.Name = 'Ref'
      | sbobj.Groups.Signals(1).Name = 'Bucket Angle'
      | sbobj.Groups.Signals(1).XData = [0 7 11 24 28.5 40 40 51.5 53.5 60]
      | sbobj.Groups.Signals(1).YData = [0 0 -90 -90 0 0 -110 -110 0 0]
      | sbobj.Groups.Signals(2).Name = 'Upper Angle'
      | sbobj.Groups.Signals(2).XData = [0 12.5 25 30 32.5 54 60]
      | sbobj.Groups.Signals(2).YData = [50 50 -20 -20 40 55 55]
      | sbobj.Groups.Signals(3).Name = 'Lower Angle'
      | sbobj.Groups.Signals(3).XData = [0 15 27.5 30 40 60]
      | sbobj.Groups.Signals(3).YData = [-60 -60 -30 -30 -60 -60]
      | sbobj.Groups.TimeRange = [0 60]
  Bucket Angle : Outport  Tag=STV Outport
  Upper Angle : Outport  Tag=STV Outport  Port=2
  Lower Angle : Outport  Tag=STV Outport  Port=3
  wires:
  Demux/3 -> Lower Angle/1
  Demux/2 -> Upper Angle/1
  FromWs/1 -> Demux/1
  Demux/1 -> Bucket Angle/1

== system Backhoe_Arm_LS/xPC Scope ==
  In1 : Inport
  "Scope (xPC) " : xpclib/Misc./Scope (xPC)   scopeno=2  scopetype=Target  autostart=on  viewmode=Graphical redraw  formatstr='%15.6f'  grid=on  ylimits=[-100, 0]  nosamples=2500  noprepostsamples=0  interleave=1  triggermode=FreeRun  triggersignal=1  trigsignalfromport=off  triggerlevel=0.0  triggerslope=Either  triggerscope=1  triggersample=0  filename=data.dat  mode=Lazy  writesize=512  autorestart=off  dynamicfilemode=off  maxwritefilesize=512*1024^2
  wires:
  In1/1 -> "Scope (xPC) "/1

== system Backhoe_Arm_LS/Arm/Bucket Assembly ==
  Bucket : Subsystem  mask(Bucket){plateSide=1.2, plateFilletR=0.2, plateDist=1.2, plateWidth=0.2, plateHoleR=0.075, bucketHeight=2, bucketLength=2, bucketThickness=0.05, bucketUpper=1.3, bucketLower=2, chordAngle=pi/6, toothLength=0.25, toothWidth=0.2, toothTip=0.025, circlePoints=45, bucketColor=yellow, bracketColor=yellow, rho=rhoSteel}
      mask prompts: plateSide "Wplate [m]"; plateFilletR "Rfillet [m]"; plateDist "Dplate [m]"; plateWidth "Tplate [m]"; plateHoleR "Rpin [m]"; bucketHeight "Hbucket [m]"; bucketLength "Wbucket [m]"; bucketThickness "Tbucket [m]"; bucketUpper "Wupper [m]"; bucketLower "Wlower [m]"; chordAngle "alpha [radians]"; toothLength "Ltooth [m]"; toothWidth "Wtooth [m]"; toothTip "Ttooth [m]"; circlePoints "Circle Mesh Resolution"; bucketColor "Bucket Color"; bracketColor "Bracket Color"; rho "Density [kg/m^3]"
      mask help:
      | Consists of the backhoe bucket assembly with attachment frame.
      |
      | Attachment points are:
      | CA: Center point of the Crank Arm link pin.
      | UA: Center Point of the Upper Arm link pin.
      | Both points are configured for Revolute joints.
      |
      | Click on Help to view a schematic of the bucket, its configurable dimension parameters and attachment points (in red).
      mask init:
      | bucketRadius = bucketHeight/(2*cos(chordAngle));
      | 
      | % Bucket Back
      | bucketBack = [];
      | % Outer wall
      | for i = 0:circlePoints;
      |    angle = (-pi/2+chordAngle) + (pi - 2*chordAngle)*(i/circlePoints);
      |    bucketBack = [bucketBack; ...
      |        (bucketRadius*cos(angle)-bucketRadius*sin(chordAngle)) ...
      |         bucketRadius*sin(angle)];
      | end
      | 
      | % Inner Wall
      | beta = acos( ( (bucketRadius*cos(chordAngle) - bucketThickness/cos(chordAngle)) ...
      |                    /(bucketRadius-bucketThickness)) );
      | for i = 0:circlePoints;
      |    angle = (pi/2 - beta) - (pi-2*beta)*(i/circlePoints);
      |    bucketBack = [bucketBack; ...
      |        ((bucketRadius-bucketThickness)*cos(angle)-bucketRadius*sin(chordAngle)) ... 
      |        (bucketRadius-bucketThickness)*sin(angle)];
      | end
      | 
      | bucketBack = [bucketBack; ...
      |               -bucketLower -(bucketHeight/2-bucketThickness);...
      |               -bucketLower -bucketHeight/2];
      |           
      | % Uncomment below to plot the cross-sections. 
      | % close all
      | % figure
      | % plot(bucketBack(:,1),bucketBack(:,2));
      mask Help: web('Backhoe_Bucket.html');
      mask Display:
      | image(imread('Backhoe_Bucket_IMAGE.png'));
      | port_label('rconn',1,'CA');
      | port_label('rconn',2,'UA');
  Crank Assembly : Subsystem  mask(Crank Assembly){LC1=1.5, WC1=0.4, TC1=0.2, DH1=1.1, RH1=0.075, LC2=1.75, WC2=0.4, TC2=0.15, DH2=1.35, RH2=0.075, DC2=0.7, Wbar=0.8, Lpin=1.3, Rpin=0.075, circlePoints=25, color1=orange, color2=darkOrange, rho1=rhoSteel, rho2=rhoSteel}
      mask prompts: LC1 "LC1 [m]"; WC1 "WC1 [m]"; TC1 "TC1 [m]"; DH1 "DH1 [m]"; RH1 "RH1 [m]"; LC2 "LC2 [m]"; WC2 "WC2 [m]"; TC2 "TC2 [m]"; DH2 "DH2 [m]"; RH2 "RH2 [m]"; DC2 "DC2 [m]"; Wbar "Upper Arm Width, Wbar [m]"; Lpin "Lpin [m]"; Rpin "Rpin [m]"; circlePoints "Circle Mesh Resolution"; color1 "Color"; color2 "Color"; rho1 "Density [kg/m^3]"; rho2 "Density [kg/m^3]"
      mask help:
      | Consists of the backhoe crank assembly that connects the upper arm and the bucket. Crank 1 attaches to either side of the upper arm linkage, and Crank 2 connects Crank 1 and the Bucket.
      |
      | Attachment points are:
      | AL: Arm attachment (Left).
      | AR: Arm attachment (Right).
      | B: Bucket attachment.
      | P: Piston attachment.
      | All attachment points are configured for Revolute joints.
      |
      | Click on Help to view a schematic of the crank assembly, its configurable dimension parameters and attachment points (in red).
      mask Help: web('Backhoe_Crank.html');
      mask Display:
      | image(imread('Backhoe_Crankassembly_IMAGE.png'));
      | port_label('rconn',1,'B');
      | port_label('rconn',2,'P');
      | port_label('lconn',1,'AL');
      | port_label('lconn',2,'AR');
  Crank to Bucket : sm_lib/Joints/Revolute Joint  SenseConstraintForceX=off  SenseConstraintForceY=off  SenseConstraintForceZ=off  SenseConstraintTorqueX=off  SenseConstraintTorqueY=off  SenseConstraintTorqueZ=off  ConstraintWrenchDir=FollowerOnBase  ConstraintWrenchFrame=BaseFrame  EquilibriumPosition=0  EquilibriumPositionUnits=deg  SpringStiffness=0  SpringStiffnessUnits=N*m/deg  DampingCoefficient=0  DampingCoefficientUnits=N*m/(deg/s)  ActuationMode=NoActuation  SensePosition=off  SenseVelocity=off  SenseAcceleration=off  SenseTorqueForce=off  PositionTargetValue=0  PositionTargetValueUnits=deg  PositionTargetSpecify=off  PositionTargetPriority=Low  VelocityTargetValue=0  VelocityTargetValueUnits=deg/s  VelocityTargetSpecify=off  VelocityTargetPriority=High  BlockFunction=simmechanics.library.joints.revolute_joint
  TAct : PMIOPort  Port=1  Side=Right
  UAL : PMIOPort  Port=2  Side=Left
  UAR : PMIOPort  Port=3  Side=Left
  UA : PMIOPort  Port=4  Side=Left
  connections:
  Bucket/RConn1 -- Crank to Bucket/RConn1
  Crank Assembly/RConn2 -- Crank to Bucket/LConn1
  Bucket/RConn2 -- UA/RConn1
  UAL/RConn1 -- Crank Assembly/LConn1
  UAR/RConn1 -- Crank Assembly/LConn2
  TAct/RConn1 -- Crank Assembly/RConn1

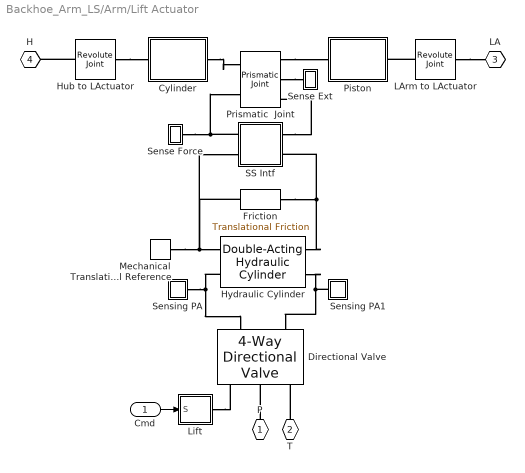
== system Backhoe_Arm_LS/Arm/Lift Actuator ==
  Cmd : Inport
  Cylinder : Subsystem
  Directional Valve : sh_lib/Valves/Directional Valves/4-Way Directional Valve  Tag=Factory Generic  mdl_type=1  area_max=hydr_valve_max_area mm^2  opening_max=hydr_valve_max_opening m  opening_tab="[  -0.002 0 0.005 0.015 ] m"  area_tab="[  1e-12 4e-12 1e-05 1.02e-05 ] m^2"  pressure_tab="[  -5e+06 -2e+06 2e+06 5e+06 ] Pa"  flow_rate_tab="[  -1e-12 -6e-14 6e+12 1e+11 ; -8e-08 -4e-08 4e+06 8e+06 ; -0.0025 -0.00103 0.001 0.0024 ; -0.00258 -0.001032 0.00106 0.00247 ; ] m^3/s"  interp_method=1  extrap_method=1  C_d=0.7  x_0_P_A=0 m  x_0_P_B=0 m  x_0_A_T=0 m  x_0_B_T=0 m  Re_cr=12  A_leak=1e-12 m^2  LocalVarLogging=[]
  Friction : fl_lib/Mechanical/Translational Elements/Translational Friction  brkwy_frc=friction_breakaway N  Col_frc=friction_coulomb N  visc_coef=friction_viscous N/(m/s)  trans_coef=10 s/m  vel_thr=1e-4 m/s  f_Log=off  v_Log=off  LocalVarNames=|f|v  LocalVarDescs=|f|v  LocalVarLogging=[0 0]
  Hub to LActuator : sm_lib/Joints/Revolute Joint  SenseConstraintForceX=off  SenseConstraintForceY=off  SenseConstraintForceZ=off  SenseConstraintTorqueX=off  SenseConstraintTorqueY=off  SenseConstraintTorqueZ=off  ConstraintWrenchDir=FollowerOnBase  ConstraintWrenchFrame=BaseFrame  EquilibriumPosition=0  EquilibriumPositionUnits=deg  SpringStiffness=0  SpringStiffnessUnits=N*m/deg  DampingCoefficient=1e1  DampingCoefficientUnits=N*m/(deg/s)  ActuationMode=NoActuation  SensePosition=off  SenseVelocity=off  SenseAcceleration=off  SenseTorqueForce=off  PositionTargetValue=-26  PositionTargetValueUnits=deg  PositionTargetSpecify=on  PositionTargetPriority=High  VelocityTargetValue=0  VelocityTargetValueUnits=deg/s  VelocityTargetSpecify=off  VelocityTargetPriority=High  BlockFunction=simmechanics.library.joints.revolute_joint
  Hydraulic Cylinder : sh_lib/Hydraulic Cylinders/Double-Acting Hydraulic Cylinder  Tag=Factory Generic  area_A=hydr_area m^2  area_B=hydr_area m^2  stroke=hydr_stroke m  init_pos=hydr_x0 m  dead_vol_A=hydr_deadvol m^3  dead_vol_B=hydr_deadvol m^3  init_pressure_A=hydr_PA0 Pa  init_pressure_B=hydr_PB0 Pa  k_sh=1.4  stiff=1e+06 N/m  D=150 N/(m/s)  or=2  LocalVarLogging=[]
  LArm to LActuator : sm_lib/Joints/Revolute Joint  SenseConstraintForceX=off  SenseConstraintForceY=off  SenseConstraintForceZ=off  SenseConstraintTorqueX=off  SenseConstraintTorqueY=off  SenseConstraintTorqueZ=off  ConstraintWrenchDir=FollowerOnBase  ConstraintWrenchFrame=BaseFrame  EquilibriumPosition=0  EquilibriumPositionUnits=deg  SpringStiffness=0  SpringStiffnessUnits=N*m/deg  DampingCoefficient=0  DampingCoefficientUnits=N*m/(deg/s)  ActuationMode=NoActuation  SensePosition=off  SenseVelocity=off  SenseAcceleration=off  SenseTorqueForce=off  PositionTargetValue=86  PositionTargetValueUnits=deg  PositionTargetSpecify=on  PositionTargetPriority=Low  VelocityTargetValue=0  VelocityTargetValueUnits=deg/s  VelocityTargetSpecify=off  VelocityTargetPriority=High  BlockFunction=simmechanics.library.joints.revolute_joint
  Lift : Subsystem
  Mechanical Translational Reference : fl_lib/Mechanical/Translational Elements/Mechanical Translational Reference  Tag=Factory Generic  f_Log=off  LocalVarNames=|f  LocalVarDescs=|f  LocalVarLogging=[]
  Piston : Subsystem
  Prismatic  Joint : sm_lib/Joints/Prismatic  Joint  SenseConstraintForceX=off  SenseConstraintForceY=off  SenseConstraintForceZ=off  SenseConstraintTorqueX=off  SenseConstraintTorqueY=off  SenseConstraintTorqueZ=off  ConstraintWrenchDir=FollowerOnBase  ConstraintWrenchFrame=BaseFrame  EquilibriumPosition=0  EquilibriumPositionUnits=m  SpringStiffness=0  SpringStiffnessUnits=N/m  DampingCoefficient=0  DampingCoefficientUnits=N/(m/s)  ActuationMode=TorqueForceActuation  SensePosition=on  SenseVelocity=on  SenseAcceleration=off  SenseTorqueForce=off  PositionTargetValue=0  PositionTargetValueUnits=m  PositionTargetSpecify=off  PositionTargetPriority=Low  VelocityTargetValue=0  VelocityTargetValueUnits=m/s  VelocityTargetSpecify=off  VelocityTargetPriority=High  BlockFunction=simmechanics.library.joints.prismatic_joint
  SS Intf : Subsystem
  Sense Ext : Subsystem
      mask Display: disp('S')
  Sense Force : Subsystem
      mask Display: disp('S')
  Sensing PA : Subsystem
      mask Display: disp('S')
  Sensing PA1 : Subsystem
      mask Display: disp('S')
  P : PMIOPort  Port=1  Side=Left
  T : PMIOPort  Port=2  Side=Left
  LA : PMIOPort  Port=3  Side=Right
  H : PMIOPort  Port=4  Side=Right
  wires:
  Cmd/1 -> Lift/1(S)
  connections:
  SS Intf/RConn1 -- Sense Force/RConn1 -- Prismatic  Joint/LConn2
  SS Intf/LConn1 -- Prismatic  Joint/RConn3
  Prismatic  Joint/RConn1 -- Piston/LConn1
  Cylinder/LConn1 -- Prismatic  Joint/LConn1
  Friction/LConn1 -- Hydraulic Cylinder/RConn1 -- SS Intf/LConn2
  Sensing PA/LConn1 -- Hydraulic Cylinder/LConn2 -- Directional Valve/LConn1
  Mechanical Translational Reference/LConn1 -- Friction/RConn1 -- SS Intf/RConn2 -- Hydraulic Cylinder/LConn1
  Hydraulic Cylinder/RConn2 -- Sensing PA1/LConn1 -- Directional Valve/LConn2
  LArm to LActuator/LConn1 -- Piston/RConn1
  LArm to LActuator/RConn1 -- LA/RConn1
  Hub to LActuator/LConn1 -- H/RConn1
  Hub to LActuator/RConn1 -- Cylinder/RConn1
  P/RConn1 -- Directional Valve/RConn2
  T/RConn1 -- Directional Valve/RConn3
  Lift/RConn1 -- Directional Valve/RConn1
  Prismatic  Joint/RConn2 -- Sense Ext/LConn1
